simulink model "sampleModel363"  (R2021b)
settings: Solver=VariableStepAuto  StartTime=0.0  StopTime=10.0  RelTol=1e-3
undefined symbols (not defined in the file or in its folder): Newton, Raphson
libraries: simulink x11
settings Model: Creator=user  LastModifiedBy=user

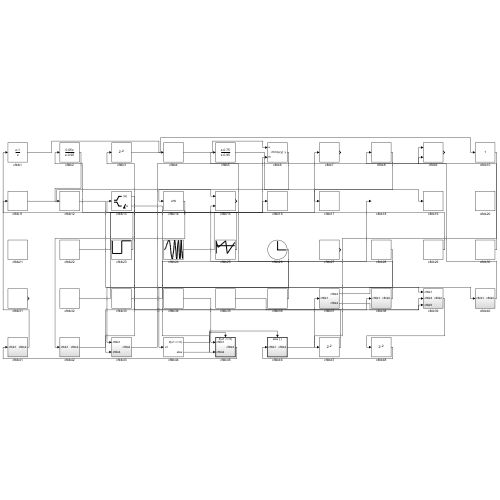
[thumbnail: Simulink's stored preview of the top-level diagram]
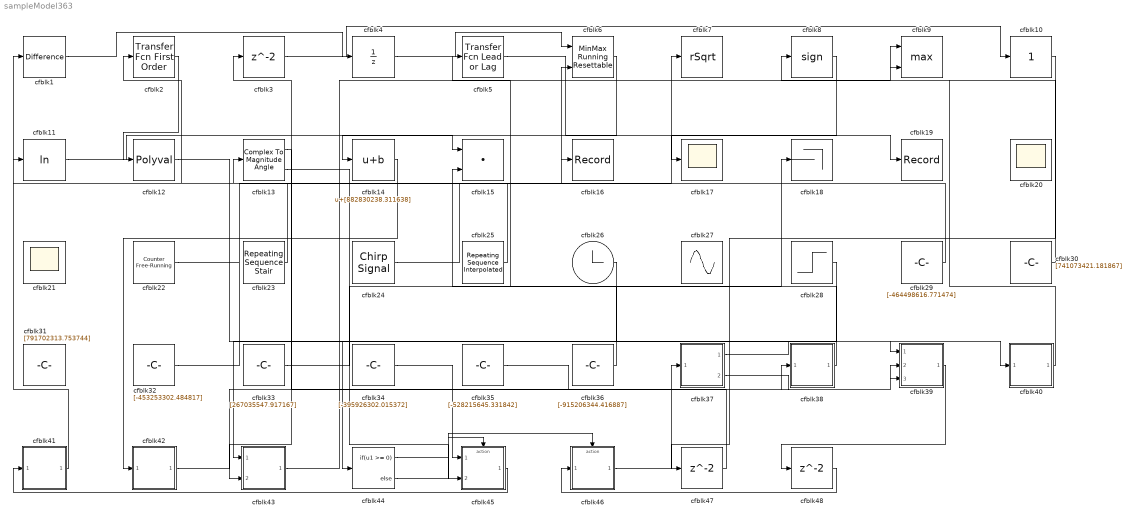
== system sampleModel363 ==
  cfblk1 : simulink/Discrete/Difference  ICPrevInput=0.0  OutMin=[]  OutMax=[]  OutDataTypeStr=Inherit: Inherit via back propagation  OutDataType=fixdt(1, 16)  OutScaling=2^-10  DoSatur=off
  cfblk10 : simulink/Math Operations/Slider Gain  gain=1  low=0  high=2
  cfblk11 : Math  Operator=log  SaturateOnIntegerOverflow=on
  cfblk12 : Polyval  Coefs=[ +2.081618890e-019, -1.441693666e-014, +4.719686976e-010, -8.536869453e-006, +1.621573104e-001, -8.087801117e+001 ]
  cfblk13 : ComplexToMagnitudeAngle
  cfblk14 : Bias  Bias=[882830238.311638]
  cfblk15 : DotProduct  InputSameDT=on  OutDataTypeStr=Inherit: Inherit via internal rule
  cfblk16 : Record  FileSettingsInternal="{\"entries\":[{\"content\":{\"excelSettings\":{\"content\":{},\"type\":\"Streamout.ExcelSettings\"}},\"type\":\"Streamout.FileSettingStorage\",\"uuid\":\"f2748134-4429-4ba9-9e65-3c862828ba1c\"}],\"packageUris\":[\"http://schema.mathworks.com/mf0/streamout_blocks/R2020a\"],\"version\":\"1.0\"}"  SignalsInternal="{\"entries\":[{\"content\":{\"signals\":[{\"content\":{\"blockPath\":[\"sampleModel363/cfblk16\"],\"channel\":[],\"dimensions\":[1],\"domain\":\"sampleModel363/cfblk16\",\"lineColor\":\"#ff6929\",\"plots\":[1],\"port\":1,\"sid\":[\"\"],\"signalID\":15014,\"signalName\":\"cfblk24\"},\"type\":\"RecordBlkView.Signal\",\"uuid\":\"2fe24df8-fca6-400d-9cc0-59fd09f53aa4\"}]},\"type\":\"RecordBlkView.InputSignals\",\"uuid\":\"2e7026b4-edde-469e-bf63-9e82d904da39\"}],\"packageUris\":[\"http://schema.mathworks.com/mf0/streamout_blocks/R2020a\"],\"version\":\"1.0\"}"  VisualizationBindings="{\"sparklinesplugin\":{\"info\":[{\"bindingParametersList\":[],\"subplotID\":1}]}}"
  cfblk17 : Scope
  cfblk18 : Terminator
  cfblk19 : Record  FileSettingsInternal="{\"entries\":[{\"content\":{\"excelSettings\":{\"content\":{},\"type\":\"Streamout.ExcelSettings\"}},\"type\":\"Streamout.FileSettingStorage\",\"uuid\":\"32a766da-25b7-45e5-be94-8c47b43e14dd\"}],\"packageUris\":[\"http://schema.mathworks.com/mf0/streamout_blocks/R2020a\"],\"version\":\"1.0\"}"  SignalsInternal="{\"entries\":[{\"content\":{\"signals\":[{\"content\":{\"blockPath\":[\"sampleModel363/cfblk19\"],\"channel\":[],\"dimensions\":[1],\"domain\":\"sampleModel363/cfblk19\",\"lineColor\":\"#139fff\",\"plots\":[1],\"port\":1,\"sid\":[\"\"],\"signalID\":15010,\"signalName\":\"cfblk5\"},\"type\":\"RecordBlkView.Signal\",\"uuid\":\"3ddf5a97-f7ba-46a7-a20f-6ed8ecc42fd7\"}]},\"type\":\"RecordBlkView.InputSignals\",\"uuid\":\"e56b51b3-d8df-4754-b99e-9f0d97b88bcc\"}],\"packageUris\":[\"http://schema.mathworks.com/mf0/streamout_blocks/R2020a\"],\"version\":\"1.0\"}"  VisualizationBindings="{\"sparklinesplugin\":{\"info\":[{\"bindingParametersList\":[],\"subplotID\":1}]}}"
  cfblk2 : simulink/Discrete/Transfer Fcn First Order  PoleZ=0.95  ICPrevOutput=0.0  DoSatur=off
  cfblk20 : Scope
      settings: Floating=on
  cfblk21 : Scope
      settings: Floating=on
  cfblk22 : simulink/Sources/Counter Free-Running  NumBits=[16.000000]  tsamp=-1
  cfblk23 : simulink/Sources/Repeating Sequence Stair  OutValues=[114831215.002136, 736007492.501561]  tsamp=-1  OutMin=[]  OutMax=[]  OutDataTypeStr=double  OutputDataTypeScalingMode=double  OutDataType=fixdt(0,8)  ConRadixGroup=Best Precision: Vector-wise  OutScaling=2^-12
  cfblk24 : simulink/Sources/Chirp Signal  f1=[772119431.049281]  T=[173109841.751595]  f2=[539200171.170052]
  cfblk25 : simulink/Sources/Repeating Sequence Interpolated  OutValues=[376281502.043075, -130510924.492913, 482252624.199647, -717076743.263491, 334243942.212013]  TimeValues=[0 0.1 0.5 0.6 1].'  LookUpMeth=Use Input Below  tsamp=0.01  OutMin=[]  OutMax=[]  OutDataTypeStr=double  OutputDataTypeScalingMode=double  OutDataType=fixdt(0,8)  OutScaling=2^-10
  cfblk26 : Clock
  cfblk27 : Sin  Amplitude=[-479213398.217903]  Bias=[459680641.918263]  SampleTime=0
  cfblk28 : Step  Time=[19.000000]  Before=[195189599.906598]  After=[-2489138.468289]  SampleTime=0
  cfblk29 : Constant  Value=[-464498616.771474]  SampleTime=1
  cfblk3 : Delay  SampleTime=1
  cfblk30 : Constant  Value=[741073421.181867]  SampleTime=1
  cfblk31 : Constant  Value=[791702313.753744]  SampleTime=1
  cfblk32 : Constant  Value=[-453253302.484817]  SampleTime=1
  cfblk33 : Constant  Value=[267035547.917167]  SampleTime=1
  cfblk34 : Constant  Value=[-395926302.015372]  SampleTime=1
  cfblk35 : Constant  Value=[-528215645.331842]  SampleTime=1
  cfblk36 : Constant  Value=[-915206344.416887]  SampleTime=1
  cfblk37 : Subsystem
  cfblk38 : Subsystem
  cfblk39 : Subsystem
  cfblk4 : UnitDelay  HasFrameUpgradeWarning=on
  cfblk40 : Subsystem
  cfblk41 : Subsystem
  cfblk42 : Subsystem
  cfblk43 : Subsystem
  cfblk44 : If  IfExpression=u1 >= 0  SampleTime=1
  cfblk45 : Subsystem  TreatAsAtomicUnit=on
  cfblk46 : Subsystem  TreatAsAtomicUnit=on
  cfblk47 : Delay  SampleTime=1
  cfblk48 : Delay  SampleTime=1
  cfblk5 : simulink/Discrete/Transfer Fcn Lead or Lag  PoleZ=0.95  ZeroZ=0.75  ICPrevOutput=0.0  ICPrevInput=0.0  DoSatur=off
      settings: SourceProductBaseCode=SL
  cfblk6 : simulink/Math Operations/MinMax Running Resettable  Function=min  vinit=0.0
  cfblk7 : Sqrt  Operator=rSqrt  AlgorithmType=Newton-Raphson  SaturateOnIntegerOverflow=on
  cfblk8 : Signum
  cfblk9 : MinMax  Function=max  Inputs=2
  wires:
  cfblk45/1(cfblk2) -> cfblk41/1(cfblk1)
  cfblk5/1 -> cfblk19/1
  cfblk4/1 -> cfblk6/1
  cfblk41/1(cfblk2) -> cfblk1/1
  cfblk14/1 -> cfblk42/1(cfblk1)
  cfblk33/1 -> cfblk18/1
  cfblk11/1 -> cfblk15/1
  cfblk26/1 -> cfblk43/1(cfblk1)
  cfblk37/1(cfblk2) -> cfblk39/1(cfblk1)
  cfblk22/1 -> cfblk7/1
  cfblk3/1 -> cfblk10/1
  cfblk30/1 -> cfblk8/1
  cfblk8/1 -> cfblk17/1
  cfblk6/1 -> cfblk14/1
  cfblk2/1 -> cfblk12/1
  cfblk40/1(cfblk2) -> cfblk9/1
  cfblk36/1 -> cfblk15/2
  cfblk32/1 -> cfblk6/2
  cfblk24/1 -> cfblk16/1
  cfblk29/1 -> cfblk11/1
  cfblk25/1 -> cfblk13/1
  cfblk23/1 -> cfblk2/1
  cfblk37/2(cfblk4) -> cfblk39/2(cfblk4)
  cfblk13/1 -> cfblk43/2(cfblk4)
  cfblk12/1 -> cfblk40/1(cfblk1)
  cfblk1/1 -> cfblk4/1
  cfblk35/1 -> cfblk39/3(cfblk5)
  cfblk28/1 -> cfblk44/1
  cfblk38/1(cfblk2) -> cfblk5/1
  cfblk43/1(cfblk2) -> cfblk9/2
  cfblk46/1(cfblk2) -> cfblk37/1(cfblk1)
  cfblk42/1(cfblk2) -> cfblk38/1(cfblk1)
  cfblk34/1 -> cfblk45/1(cfblk1)
  cfblk13/2 -> cfblk45/2(cfblk4)
  cfblk44/1 -> cfblk45/Action
  cfblk44/2 -> cfblk46/Action
  cfblk10/1 -> cfblk47/1
  cfblk47/1 -> cfblk3/1
  cfblk39/1(cfblk2) -> cfblk48/1
  cfblk48/1 -> cfblk46/1(cfblk1)

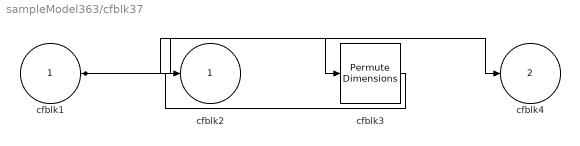
== system sampleModel363/cfblk37 ==
  cfblk1 : Inport
  cfblk3 : PermuteDimensions
  cfblk2 : Outport
  cfblk4 : Outport  Port=2
  wires:
  cfblk1/1 -> cfblk4/1, cfblk3/1
  cfblk3/1 -> cfblk2/1

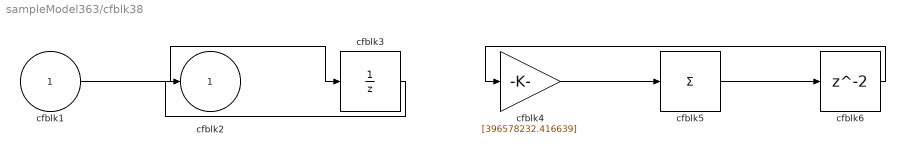
== system sampleModel363/cfblk38 ==
  cfblk1 : Inport
  cfblk3 : UnitDelay  HasFrameUpgradeWarning=on
  cfblk4 : Gain  Gain=[396578232.416639]
  cfblk5 : Sum  Inputs=+
  cfblk6 : Delay  SampleTime=1
  cfblk2 : Outport
  wires:
  cfblk1/1 -> cfblk3/1
  cfblk4/1 -> cfblk5/1
  cfblk3/1 -> cfblk2/1
  cfblk5/1 -> cfblk6/1
  cfblk6/1 -> cfblk4/1

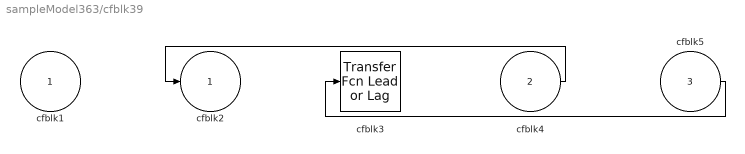
== system sampleModel363/cfblk39 ==
  cfblk1 : Inport
  cfblk4 : Inport  Port=2
  cfblk5 : Inport  Port=3
  cfblk3 : simulink/Discrete/Transfer Fcn Lead or Lag  PoleZ=0.95  ZeroZ=0.75  ICPrevOutput=0.0  ICPrevInput=0.0  DoSatur=off
      settings: SourceProductBaseCode=SL
  cfblk2 : Outport
  wires:
  cfblk4/1 -> cfblk2/1
  cfblk5/1 -> cfblk3/1

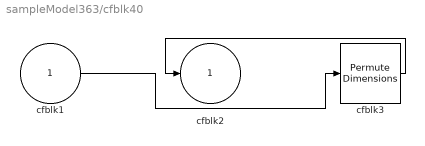
== system sampleModel363/cfblk40 ==
  cfblk1 : Inport
  cfblk3 : PermuteDimensions
  cfblk2 : Outport
  wires:
  cfblk3/1 -> cfblk2/1
  cfblk1/1 -> cfblk3/1

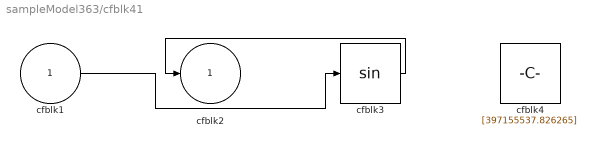
== system sampleModel363/cfblk41 ==
  cfblk1 : Inport
  cfblk3 : Trigonometry
  cfblk4 : Constant  Value=[397155537.826265]  SampleTime=1
  cfblk2 : Outport
  wires:
  cfblk3/1 -> cfblk2/1
  cfblk1/1 -> cfblk3/1

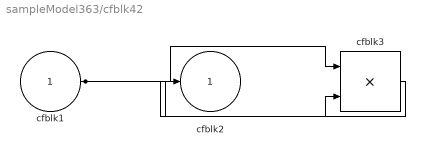
== system sampleModel363/cfblk42 ==
  cfblk1 : Inport
  cfblk3 : Product  Inputs=**
  cfblk2 : Outport
  wires:
  cfblk1/1 -> cfblk3/1, cfblk3/2
  cfblk3/1 -> cfblk2/1

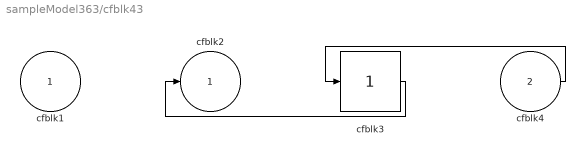
== system sampleModel363/cfblk43 ==
  cfblk1 : Inport
  cfblk4 : Inport  Port=2
  cfblk3 : simulink/Math Operations/Slider Gain  gain=1  low=0  high=2
  cfblk2 : Outport
  wires:
  cfblk4/1 -> cfblk3/1
  cfblk3/1 -> cfblk2/1

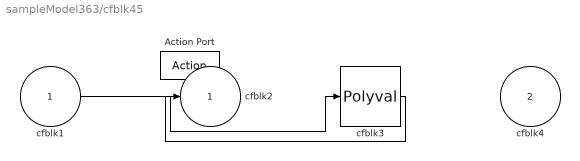
== system sampleModel363/cfblk45 ==
  cfblk1 : Inport
  cfblk4 : Inport  Port=2
  Action Port : ActionPort  ActionPortLabel=if(u1 >= 0)
  cfblk3 : Polyval  Coefs=[ +2.081618890e-019, -1.441693666e-014, +4.719686976e-010, -8.536869453e-006, +1.621573104e-001, -8.087801117e+001 ]
  cfblk2 : Outport
  wires:
  cfblk1/1 -> cfblk3/1
  cfblk3/1 -> cfblk2/1

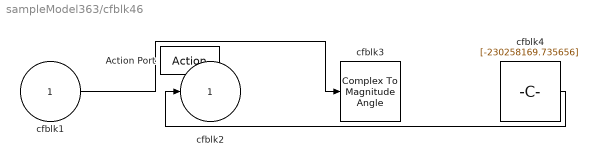
== system sampleModel363/cfblk46 ==
  cfblk1 : Inport
  Action Port : ActionPort  ActionPortLabel=else
  cfblk3 : ComplexToMagnitudeAngle
  cfblk4 : Constant  Value=[-230258169.735656]  SampleTime=1
  cfblk2 : Outport
  wires:
  cfblk4/1 -> cfblk2/1
  cfblk1/1 -> cfblk3/1
